simulink model "GA_z"  (R2024a)
settings: Solver=FixedStepAuto  StartTime=0.0  StopTime=250  FixedStep=1e-3  RelTol=1e-3
InitFcn:
  | % close;
  | % % % z
  | k_p_z = -4;
  | k_i_z = -.5;
  | k_d_z = -8;
  | k_a_z = -2;
  | % %
  | % % % psi
  | k_p_psi = 5.8;
  | k_i_psi = 0;
  | k_d_psi = .8;
  | k_a_psi = 0;
  | % %
  | % % phi
  | k_p_phi = 1;
  | k_d_phi = .3;
  | %
  | % % tt
  | k_p_tt = 1;
  | k_d_tt = .3;
  | %
  | % % x
  | k_p_x = -5.99;
  | k_i_x = -2.8;
  | k_d_x = -1.244;
  | k_a_x = -7.94;
  | %
  | % % y
  | k_p_y = 5.99;
  | k_i_y = 2.8;
  | k_d_y = 1.244;
  | k_a_y = 7.94;
StopFcn:
  | plot3(x,y,-z,['b','-'],x_g,y_g,-z_g,['r','--'],'LineWidth',1.25);
  | xlabel('x');
  | ylabel('y');
  | zlabel('z');
  | grid on;
undefined symbols (not defined in the file): k_a_phi, k_a_tt, k_i_phi, k_i_tt
libraries: simulink x6
settings Model: Creator=luand  LastModifiedBy=luand
settings DataIOCC: ReturnWorkspaceOutputs=off

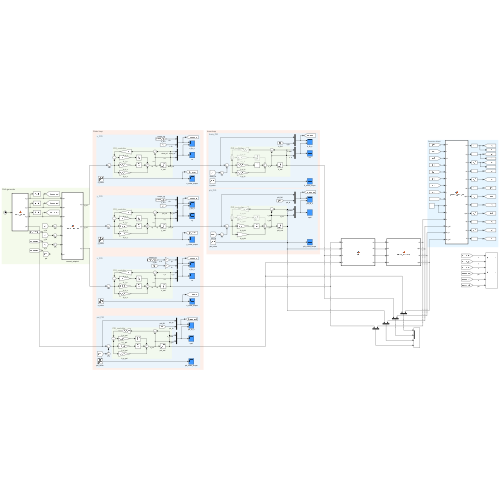
[thumbnail: Simulink's stored preview of the top-level diagram]
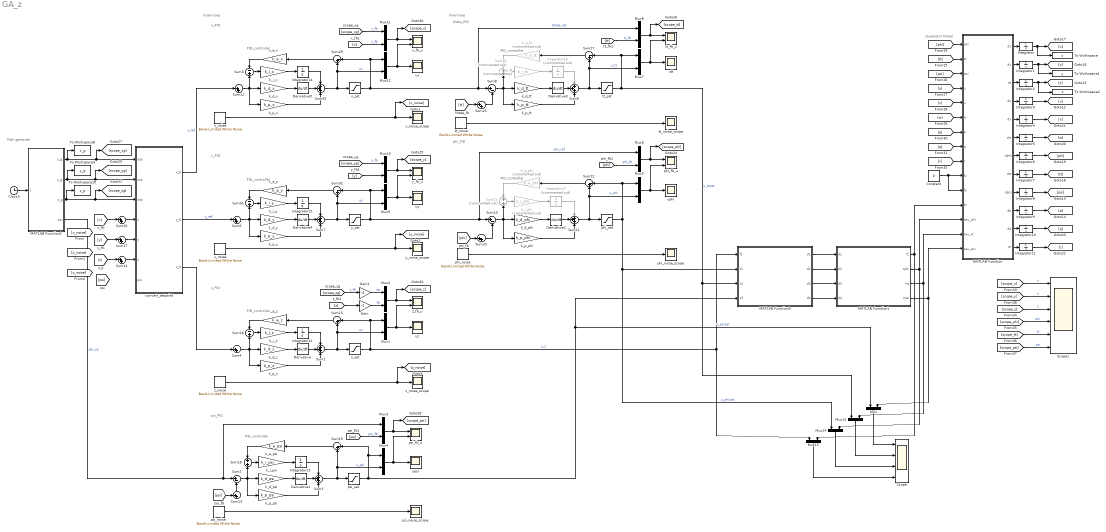
== system GA_z ==
  note: Path generate
  note: Inner loop
  note: z_PID
  note: PID_controller
  note: PID_controller
  note: psi_PID
  note: Quadrotor Model
  note: PID_controller
  note: PID_controller
  note: PID_controller
  note: PID_controller
  note: theta_PID
  note: phi_PID
  note: Outer loop
  note: y_PID
  note: x_PID
  Clock5 : Clock
  Constant : Constant  Value=0
  Derivative{,1..5} (6 alike) : Derivative
  Gain : Gain  Gain=-1
  Gain1 : Gain  Gain=-1
  Integrator{,1,3..5} (5 alike) : Integrator  LimitOutput=on  UpperSaturationLimit=10000  LowerSaturationLimit=-10000
  Integrator10 : Integrator  LimitOutput=on  UpperSaturationLimit=100  LowerSaturationLimit=-100
  Integrator11 : Integrator  LimitOutput=on  UpperSaturationLimit=100  LowerSaturationLimit=-100
  Integrator{6..8,12..15} (7 alike) : Integrator  LimitOutput=on  UpperSaturationLimit=1000  LowerSaturationLimit=-1000
  Integrator16 : Integrator  Commented=on
  Integrator17 : Integrator  Commented=on  LimitOutput=on  UpperSaturationLimit=1000  LowerSaturationLimit=-1000
  Integrator2 : Integrator  LimitOutput=on  UpperSaturationLimit=0  LowerSaturationLimit=-1000
  Integrator9 : Integrator  LimitOutput=on  UpperSaturationLimit=100  LowerSaturationLimit=-100
  MATLAB Function : MATLAB Function  TreatAsAtomicUnit=on
  MATLAB Function1 : MATLAB Function  TreatAsAtomicUnit=on
  MATLAB Function2 : MATLAB Function  TreatAsAtomicUnit=on
  MATLAB Function3 : MATLAB Function  TreatAsAtomicUnit=on
  Mux{,1..15} (16 alike) : Mux  Inputs=2
  Scope : Scope  NumInputPorts=4
  Scope1 : Scope  NumInputPorts=6
  Sum{1,3,7,9,11,33} (6 alike) : Sum  Inputs=+++
  Sum10 : Sum  Inputs=|+-
  Sum{4,6,12,14,17,20,23,25} (8 alike) : Sum  Inputs=|++
  Sum13 : Sum  Inputs=++|
  Sum{15,19,22,27,29,32} (6 alike) : Sum  Inputs=|-+
  Sum16 : Sum  Inputs=-|+
  Sum18 : Sum  Inputs=+|+
  Sum2 : Sum  Inputs=|+-
  Sum21 : Sum  Commented=on  Inputs=+|+
  Sum26 : Sum  Commented=on  Inputs=+|+
  Sum31 : Sum  Inputs=-|+
  Sum5 : Sum  Inputs=-|+
  Sum8 : Sum  Inputs=|+-
  To Workspace : ToWorkspace  VariableName=x  SampleTime=-1
      settings: Save2DSignal=2-D array (concatenate along first dimension)
  To Workspace1 : ToWorkspace  VariableName=y  SampleTime=-1
      settings: Save2DSignal=2-D array (concatenate along first dimension)
  To Workspace10 : ToWorkspace  VariableName=z_g  SampleTime=-1
      settings: Save2DSignal=2-D array (concatenate along first dimension)
  To Workspace2 : ToWorkspace  VariableName=z  SampleTime=-1
      settings: Save2DSignal=2-D array (concatenate along first dimension)
  To Workspace8 : ToWorkspace  VariableName=x_g  SampleTime=-1
      settings: Save2DSignal=2-D array (concatenate along first dimension)
  To Workspace9 : ToWorkspace  VariableName=y_g  SampleTime=-1
      settings: Save2DSignal=2-D array (concatenate along first dimension)
  convert_setpoint : MATLAB Function  TreatAsAtomicUnit=on
  k_a_phi : Gain  Commented=on  Gain=k_a_phi
  k_a_psi : Gain  Gain=k_a_psi
  k_a_tt : Gain  Commented=on  Gain=k_a_tt
  k_a_x : Gain  Gain=k_a_x
  k_a_y : Gain  Gain=k_a_y
  k_a_z : Gain  Gain=k_a_z
  k_d_phi : Gain  Gain=k_d_phi
  k_d_psi : Gain  Gain=k_d_psi
  k_d_tt : Gain  Gain=k_d_tt
  k_d_x : Gain  Gain=k_d_x
  k_d_y : Gain  Gain=k_d_y
  k_d_z : Gain  Gain=k_d_z
  k_i_phi : Gain  Commented=on  Gain=k_i_phi
  k_i_psi : Gain  Gain=k_i_psi
  k_i_tt : Gain  Commented=on  Gain=k_i_tt
  k_i_x : Gain  Gain=k_i_x
  k_i_y : Gain  Gain=k_i_y
  k_i_z : Gain  Gain=k_i_z
  k_p_phi : Gain  Gain=k_p_phi
  k_p_psi : Gain  Gain=k_p_psi
  k_p_tt : Gain  Gain=k_p_tt
  k_p_x : Gain  Gain=k_p_x
  k_p_y : Gain  Gain=k_p_y
  k_p_z : Gain  Gain=k_p_z
  phi_fb_u : Scope  NumInputPorts=2
  phi_noise : simulink/Sources/Band-Limited White Noise  Cov=[0.001]  Ts=1  seed=[23341]
  phi_noise_scope : Scope
  phi_sat : Saturate  UpperLimit=100  LowerLimit=-100
  psi_fb_u : Scope  NumInputPorts=2
  psi_noise : simulink/Sources/Band-Limited White Noise  Cov=[0.0005]  Ts=1  seed=[12424]
  psi_noise_scope : Scope
  psi_sat : Saturate  UpperLimit=50  LowerLimit=-50
  tt_fb_u : Scope  NumInputPorts=2
  tt_noise : simulink/Sources/Band-Limited White Noise  Cov=[0.001]  Ts=1  seed=[23341]
  tt_noise_scope : Scope
  tt_sat : Saturate  UpperLimit=100  LowerLimit=-100
  uphi : Scope
  upsi : Scope
  utt : Scope
  ux : Scope
  uy : Scope
  uz : Scope
  x_fb_u : Scope  NumInputPorts=2
  x_noise : simulink/Sources/Band-Limited White Noise  Cov=[0.0001]  Ts=1  seed=[23341]
  x_noise_scope : Scope
  x_sat : Saturate  UpperLimit=pi/15  LowerLimit=-pi/15
  y_fb_u : Scope  NumInputPorts=2
  y_noise : simulink/Sources/Band-Limited White Noise  Cov=[0.0001]  Ts=1  seed=[24432]
  y_noise_scope : Scope
  y_sat : Saturate  UpperLimit=pi/15  LowerLimit=-pi/15
  z_fb_u : Scope  NumInputPorts=2
  z_noise : simulink/Sources/Band-Limited White Noise  Cov=[0.01]  Ts=1  seed=[55123]
  z_noise_scope : Scope
  z_sat : Saturate  UpperLimit=40  LowerLimit=0
  wires:
  k_a_phi/1 -> Sum21/1
  [phi] -> Sum23/1
  Sum23/1 -> Sum10/2
  Sum11/1 -> Mux5/2, Sum22/2, phi_sat/1  "u_phi"
  k_d_phi/1 -> Derivative2/1
  [phi] -> Mux6/2  "phi_fb"
  Mux5/1 -> uphi/1, phi_fb_u/2
  Mux6/1 -> phi_fb_u/1, [scope_phi]
  x_sat/1 -> Mux12/1, Sum29/1, Mux8/1, Sum8/1  "theta_ref"
  Sum21/1 -> k_i_phi/1
  [r] -> MATLAB Function/9(r)
  MATLAB Function2/4(psi) -> Mux3/1, Sum2/1  "psi_sp"
  phi_noise/1 -> phi_noise_scope/1
  Integrator8/1 -> [psi]
  Sum13/1 -> Sum2/2
  Sum19/1 -> k_a_psi/1
  [psi] -> Mux3/2  "psi_fb"
  MATLAB Function/11(dq) -> Integrator10/1
  Mux4/1 -> upsi/1, psi_fb_u/2
  Constant/1 -> MATLAB Function/11(fy), MATLAB Function/10(fx)
  k_a_psi/1 -> Sum18/1
  Mux1/1 -> uz/1, z_fb_u/2
  Mux3/1 -> [scope_psi], psi_fb_u/1
  k_p_psi/1 -> Sum3/3
  Derivative1/1 -> Sum3/2
  Gain/1 -> Mux2/2  "fb"
  Integrator5/1 -> [w]
  [tt] -> MATLAB Function/2(tt)
  Sum22/1 -> k_a_phi/1
  k_p_phi/1 -> Sum11/3
  Integrator/1 -> To Workspace/1, [x]
  psi_sat/1 -> MATLAB Function3/4(t3), Mux/1, Sum19/1, Mux4/1  "u_psisat"
  MATLAB Function/4(du) -> Integrator3/1
  k_d_psi/1 -> Derivative1/1
  Sum16/1 -> k_i_z/1
  Integrator12/1 -> Sum1/1
  k_a_z/1 -> Sum16/1
  Mux2/1 -> [scope_z], z_fb_u/1
  [phi] -> MATLAB Function/1(phi)
  k_d_z/1 -> Derivative/1
  z_noise/1 -> [z_noise], z_noise_scope/1
  Integrator10/1 -> [q]
  k_i_z/1 -> Integrator12/1
  Sum1/1 -> Sum15/2, Mux1/2, z_sat/1  "uz"
  [psi] -> Sum13/1
  Sum18/1 -> k_i_psi/1
  Derivative2/1 -> Sum11/2
  [psi] -> MATLAB Function/3(psi)
  k_i_phi/1 -> Integrator17/1
  phi_sat/1 -> MATLAB Function3/2(t1), Mux14/1, Mux5/1, Sum22/1  "u_phisat"
  k_i_tt/1 -> Integrator16/1
  k_i_y/1 -> Integrator15/1
  z_sat/1 -> Mux15/1, MATLAB Function3/1(fz), Mux1/1, Sum15/1  "u_z"
  [p] -> MATLAB Function/7(p)
  MATLAB Function/1(dx) -> Integrator/1
  Integrator7/1 -> [tt]
  Sum2/1 -> Sum18/2, k_d_psi/1, k_p_psi/1
  Integrator1/1 -> To Workspace1/1, [y]
  MATLAB Function/2(dy) -> Integrator1/1
  k_i_psi/1 -> Integrator13/1
  Integrator3/1 -> [u]
  Sum3/1 -> psi_sat/1, Mux4/2, Sum19/2  "u_psi"
  Integrator2/1 -> To Workspace2/1, [z]
  [w] -> MATLAB Function/6(w)
  Integrator11/1 -> [r]
  Integrator9/1 -> [p]
  [u] -> MATLAB Function/4(u)
  Integrator6/1 -> [phi]
  MATLAB Function/5(dv) -> Integrator4/1
  psi_noise/1 -> psi_noise_scope/1
  MATLAB Function/6(dw) -> Integrator5/1
  [z] -> Gain/1
  Integrator4/1 -> [v]
  MATLAB Function/12(dr) -> Integrator11/1
  MATLAB Function/9(dpsi) -> Integrator8/1
  [q] -> MATLAB Function/8(q)
  Sum10/1 -> k_d_phi/1, Sum21/2, k_p_phi/1
  [v] -> MATLAB Function/5(v)
  MATLAB Function/10(dp) -> Integrator9/1
  MATLAB Function/8(dtt) -> Integrator7/1
  Sum15/1 -> k_a_z/1
  MATLAB Function/3(dz) -> Integrator2/1
  MATLAB Function/7(dphi) -> Integrator6/1
  Integrator17/1 -> Sum11/1
  [tt] -> Sum25/1
  Sum25/1 -> Sum8/2
  Integrator16/1 -> Sum9/1
  k_p_tt/1 -> Sum9/3
  Sum26/1 -> k_i_tt/1
  k_d_tt/1 -> Derivative3/1
  Derivative3/1 -> Sum9/2
  k_a_tt/1 -> Sum26/1
  Sum27/1 -> k_a_tt/1
  tt_sat/1 -> MATLAB Function3/3(t2), Mux13/1, Mux7/1, Sum27/1  "u_ttsat"
  y_sat/1 -> Mux9/1, Sum32/1, Mux6/1, Sum10/1  "phi_ref"
  Mux8/1 -> [scope_tt], tt_fb_u/1
  Mux7/1 -> utt/1, tt_fb_u/2
  [tt] -> Mux8/2  "tt_fb"
  Sum9/1 -> Mux7/2, Sum27/2, tt_sat/1  "u_tt"
  tt_noise/1 -> tt_noise_scope/1
  Sum8/1 -> k_d_tt/1, Sum26/2, k_p_tt/1
  Integrator13/1 -> Sum3/1
  Clock5/1 -> MATLAB Function2/1(t)
  k_d_y/1 -> Derivative4/1
  Integrator15/1 -> Sum7/1
  k_p_y/1 -> Sum7/3
  Sum31/1 -> k_i_y/1
  k_a_y/1 -> Sum31/1
  Sum7/1 -> Mux9/2, Sum32/2, y_sat/1  "uy"
  Sum32/1 -> k_a_y/1
  y_noise/1 -> [y_noise], y_noise_scope/1
  x_noise/1 -> [x_noise], x_noise_scope/1
  Sum29/1 -> k_a_x/1
  Sum33/1 -> x_sat/1, Sum29/2, Mux12/2  "ux"
  k_a_x/1 -> Sum5/1
  Sum5/1 -> k_i_x/1
  k_p_x/1 -> Sum33/3
  Integrator14/1 -> Sum33/1
  k_d_x/1 -> Derivative5/1
  k_i_x/1 -> Integrator14/1
  [y] -> Mux10/2
  Mux10/1 -> [scope_y], y_fb_u/1
  Mux9/1 -> uy/1, y_fb_u/2
  Mux11/1 -> x_fb_u/1, [scope_x]
  Mux12/1 -> ux/1, x_fb_u/2
  [x] -> Mux11/2  "x_fb"
  [scope_x] -> Scope1/1  "x"
  [scope_y] -> Scope1/2  "y"
  [scope_z] -> Scope1/3  "z"
  [scope_psi] -> Scope1/6  "psi"
  [scope_phi] -> Scope1/4  "phi"
  [scope_tt] -> Scope1/5  "tt"
  Derivative4/1 -> Sum7/2
  Derivative5/1 -> Sum33/2
  MATLAB Function2/1(x_g) -> convert_setpoint/1(xsp), [scope_xg], To Workspace8/1
  MATLAB Function2/2(y_g) -> [scope_yg], convert_setpoint/2(ysp), To Workspace9/1
  MATLAB Function2/3(z_g) -> convert_setpoint/3(zsp), [scope_zg], To Workspace10/1
  Sum4/1 -> Sum16/2, k_p_z/1, k_d_z/1
  Sum12/1 -> Sum5/2, k_p_x/1, k_d_x/1
  convert_setpoint/2(y_b) -> Sum6/1  "y_ref"
  Sum6/1 -> Sum31/2, k_p_y/1, k_d_y/1
  k_p_z/1 -> Sum1/3
  Derivative/1 -> Sum1/2
  Gain1/1 -> Mux2/1  "sp"
  convert_setpoint/3(z_b) -> Sum4/1
  [scope_zg] -> Gain1/1  "x_fb"
  [scope_yg] -> Mux10/1  "x_fb"
  [scope_xg] -> Mux11/1  "x_fb"
  convert_setpoint/1(x_b) -> Sum12/1  "x_ref"
  [z] -> Sum14/1
  Sum14/1 -> convert_setpoint/6(z)
  Sum17/1 -> convert_setpoint/5(y)
  [y] -> Sum17/1
  [x] -> Sum20/1
  Sum20/1 -> convert_setpoint/4(x)
  MATLAB Function3/1(d1) -> MATLAB Function1/1(d1)
  MATLAB Function3/2(d2) -> MATLAB Function1/2(d2)
  MATLAB Function3/3(d3) -> MATLAB Function1/3(d3)
  MATLAB Function3/4(d4) -> MATLAB Function1/4(d4)
  Mux/1 -> Scope/1
  Mux13/1 -> Scope/2
  Mux14/1 -> Scope/3
  Mux15/1 -> Scope/4
  MATLAB Function1/1(fz) -> MATLAB Function/12(fz), Mux15/2
  MATLAB Function1/2(tphi) -> MATLAB Function/13(tau_phi), Mux14/2
  MATLAB Function1/3(ttt) -> MATLAB Function/14(tau_tt), Mux13/2
  MATLAB Function1/4(tpsi) -> Mux/2, MATLAB Function/15(tau_psi)

== matlab function GA_z/MATLAB Function3 ==
  data: d1 output; d2 output; d3 output; d4 output; fz input; t1 input; t2 input; t3 input
function [d1,d2,d3,d4] = M(fz,t1,t2,t3)

fz = fz+200;

d1=4.7438*fz + 33.3333*t1 + -33.3333*t2 + 41.6667*t3;
if (d1<0) 
    d1=0; 
end
if (d1>10000)
    d1=10000;
end
d1=sqrt(d1);

d2=4.7438*fz + -33.3333*t1 + -33.3333*t2 + -41.6667*t3;
if (d2<0)
    d2=0;
end
if (d2>10000)
    d2=10000;
end
d2=sqrt(d2);

d3=4.7438*fz + 33.3333*t1 + 33.3333*t2 + -41.6667*t3;
if (d3<0)
    d3=0;
end
if (d3>10000)
    d3=10000;
end
d3=sqrt(d3);

d4=4.7438*fz + -33.3333*t1 + 33.3333*t2 + 41.6667*t3;
if (d4<0)
    d4=0;
end
if (d4>10000) 
    d4=10000;
end
d4=sqrt(d4);

== matlab function GA_z/MATLAB Function1 ==
  data: fz output; tphi output; ttt output; tpsi output; d1 input; d2 input; d3 input; d4 input
function [fz,tphi,ttt,tpsi] = Motor_dynamics(d1,d2,d3,d4)

d1=d1*d1;
d2=d2*d2;
d3=d3*d3;
d4=d4*d4;

fz=0.05*(d1+d2+d3+d4)-200;
tphi=0.0075*(d1-d2+d3-d4);
ttt=.0075*(-d1-d2+d3+d4);
tpsi=.006*(d1-d2-d3+d4);

== matlab function GA_z/MATLAB Function ==
  data: phi input; tt input; psi input; u input; dx output; v input; w input; p input; q input; r input; fx input; fy input; fz input; tau_phi input; tau_tt input; tau_psi input; dy output; dz output; du output; dv output; dw output; dphi output; dtt output; dpsi output; dp output; dq output; dr output
function [dx,dy,dz,du,dv,dw,dphi,dtt,dpsi,dp,dq,dr]=Dynamics_plustype(phi,tt,psi,u,v,w,p,q,r,fx,fy,fz,tau_phi,tau_tt,tau_psi)

% Eqs. 16-19

M = 1.2;
m = .075;
g = 9.81;
R = .1;
l = .22;

Jx = .4*M*R*R+2*l*l*m;
Jy = .4*M*R*R+2*l*l*m;
Jz = .4*M*R*R+4*l*l*m;

dx = cos(tt)*cos(psi)*u+(sin(phi)*sin(tt)*cos(psi)-cos(phi)*sin(psi))*v+(cos(phi)*sin(tt)*cos(psi)+sin(phi)*sin(psi))*w;
dy = cos(tt)*sin(psi)*u+(sin(phi)*sin(tt)*sin(psi)+cos(phi)*cos(psi))*v+(cos(phi)*sin(tt)*sin(psi)-sin(phi)*cos(psi))*w;
dz = -(sin(tt)*u-sin(phi)*cos(tt)*v-cos(phi)*cos(tt)*w);

du = (r*v-q*w)-g*sin(tt);
dv = (p*w-r*u)+g*cos(tt)*sin(phi);
dw = (q*u-p*v)+g*cos(tt)*cos(phi)-fz/(M+4*m);

dphi = p+sin(phi)*tan(phi)*q+cos(phi)*tan(tt)*r;
dtt  = cos(phi)*q-sin(phi)*r;
dpsi = sin(phi)*q/cos(tt)+cos(phi)*r/cos(tt);

dp = ((Jy-Jz)*q*r+tau_phi)/Jx;
dq = ((Jz-Jx)*p*r+tau_tt)/Jy;
dr = ((Jx-Jy)*q*p+tau_psi)/Jz;

== matlab function GA_z/MATLAB Function2 ==
  data: t input; x_g output; y_g output; z_g output; psi output
function [x_g,y_g,z_g,psi] = path_ground(t)

% psi = 100-100*exp(-.02*t);
psi = 0;
% psi = sin(.05*t);
% psi = t/2;

% x_g=0;
% y_g=0;
% if t<30
%     z_g = -10;
% elseif t<70
%     z_g = -20;
% elseif t<100
%     z_g = -30;
% else
%     z_g = 0;
% end

A = 10; % x range
a = 5; % grid x
B = 10; % y range
b = 4; % grid y
C = 10;% z range 
coef = .07;
x_g = (A-.2*exp(-.014*(t-279.4)))*cos(a*coef*t);
y_g = (B-.2*exp(-.014*(t-279.4)))*sin(b*coef*t);
z_g = -C*(1-exp(-5*coef*t));%+5*sin(.3*t);

% A = 20; % x range
% a = 2; % grid x
% B = 20; % y range
% b = 2; % grid y
% C = 10;% z range 
% coef = .07;
% x_g = (10-.2*exp(-.014*(t-279.4)))*cos(a*coef*t);
% y_g = (10-.2*exp(-.014*(t-279.4)))*sin(b*coef*t);
% z_g = -10; % dont know why step Z work
% z_g = -(10-.2*exp(-.014*(t-279.4)));
% z_g = -(10-10*exp(-.05*t));

% if t<25
%     x_g = 1*t/25;
%     y_g = 1*t/25;
%     z_g = -3-2*t/25;
% elseif t<50
%     x_g = 1+(t-25)/25;
%     y_g = 1;
%     z_g = -5-2*(t-25)/25;
% elseif t<75
%     x_g = 2;
%     y_g = 1+(t-50)/25;
%     z_g = -7-2*(t-50)/25;
% elseif t<100
%     x_g = 2-3*(t-75)/25;
%     y_g = 2+(t-75)/25;
%     z_g = -9-2*(t-75)/25;
% elseif t<125
%     x_g = -1;
%     y_g = 3-4*(t-100)/25;
%     z_g = -11-2*(t-100)/25;
% elseif t<150
%     x_g = -1+4*(t-125)/25;
%     y_g = -1;
%     z_g = -13-2*(t-125)/25;
% elseif t<175
%     x_g = 3-2*(t-150)/25;
%     y_g = -1+5*(t-150)/25;
%     z_g = -15-2*(t-150)/25;
% else
%     x_g = 1-min(1,1*(t-175)/25);
%     y_g = 4-min(4,4*(t-175)/25);
%     z_g = -17+min(16,16*(t-175)/25);
% end

% if t<50
%     a=2*exp(.05*(t-50));
%     b=2;
% elseif t<100
%     a=2+exp(.05*(t-100));
%     b=3;
% elseif t<150
%     a=3+exp(.05*(t-150));
%     b=4;
% else
%     b=4*(exp(.02*(150-t)));
%     a=4+4*exp(.1*(t-200));
% end
% z_g = min(-5,-5*b);
% x_g = a*cos(.5*t);
% y_g = a*sin(.5*t);

== matlab function GA_z/convert_setpoint ==
  data: xsp input; x_b output; y_b output; ysp input; zsp input; x input; y input; z input; psi input; z_b output
% Ground setpoint to body
function [x_b,y_b,z_b] = convert_setpoint(xsp,ysp,zsp,x,y,z,psi)
xyz_sp_g = [xsp ysp zsp 1];

% R_body_to_ground = [cos(psi)*cos(theta) cos(psi)*sin(theta)*sin(phi)-sin(psi)*cos(phi) cos(psi)*sin(theta)*cos(phi)+sin(psi)*sin(phi);
%                     sin(psi)*cos(theta) sin(psi)*sin(theta)*sin(phi)+cos(psi)*cos(phi) sin(psi)*sin(theta)*cos(phi)-cos(psi)*sin(phi);
%                     -sin(theta) cos(theta)*sin(phi) cos(theta)*cos(phi)];
% P_body_to_ground = [x y z]';
% % T_body_to_ground = [R_body_to_ground P_body_to_ground; 0 0 0 1];
% 
% P_ground_to_body = [-P_body_to_ground'*R_body_to_ground(:,1);
%                     -P_body_to_ground'*R_body_to_ground(:,2);
%                     -P_body_to_ground'*R_body_to_ground(:,3)];
% T_ground_to_body = [R_body_to_ground' P_ground_to_body; 0 0 0 1];
% 
% xyz_sp_b = T_ground_to_body*xyz_sp_g';
% 
% x_b = xyz_sp_b(1);
% y_b = xyz_sp_b(2);
% z_b = xyz_sp_b(3);

R_body_to_ground = [cos(psi) -sin(psi) 0;
                    sin(psi) cos(psi) 0;
                    0 0 1];
P_body_to_ground = [x y z];
P_ground_to_body = [-P_body_to_ground*R_body_to_ground(:,1);
                    -P_body_to_ground*R_body_to_ground(:,2);
                    -P_body_to_ground*R_body_to_ground(:,3)];
T_ground_to_body = [R_body_to_ground' P_ground_to_body; 0 0 0 1];
xyz_sp_b = T_ground_to_body*xyz_sp_g';

x_b = xyz_sp_b(1);
y_b = xyz_sp_b(2);
z_b = xyz_sp_b(3);
